simulink model "BLIMP_DYNAMICS_MODEL_HOLD"  (R2024b)
settings: Solver=VariableStepAuto  StartTime=0.0  StopTime=240  RelTol=1e-3
values from neighbouring files (symbols this model uses):
  A_alt_aug = [A_alt, zeros(size(A_alt,1),1); -C_alt, 0]    [ALTITUDE_DYNAMICS.m]
  A_fwd_aug = [A_fwd, zeros(size(A_fwd,1),1); -C_fwd, 0]    [FORWARD_DYNAMICS.m]
  A_rot_aug = [A_rot, zeros(size(A_rot,1),1); -C_rot, 0]    [ROTATIONAL_DYNAMICS.m]
  B_alt_aug = [B_alt; 0]    [ALTITUDE_DYNAMICS.m]
  B_fwd_aug = [B_fwd; 0]    [FORWARD_DYNAMICS.m]
  B_rot_aug = [B_rot; 0]    [ROTATIONAL_DYNAMICS.m]
  C_alt_aug = [C_alt 0]    [ALTITUDE_DYNAMICS.m]
  C_fwd_aug = [C_fwd 0]    [FORWARD_DYNAMICS.m]
  C_rot_aug = [C_rot 0]    [ROTATIONAL_DYNAMICS.m]
  D_alt_aug = D_alt    [ALTITUDE_DYNAMICS.m]
  D_fwd_aug = D_fwd    [FORWARD_DYNAMICS.m]
  D_rot_aug = D_rot    [ROTATIONAL_DYNAMICS.m]
  INIT_COND_alt = [0, 0, 0, 0]    [ALTITUDE_DYNAMICS.m]
  INIT_COND_fwd = [0, 0, 100, 0, 0]    [FORWARD_DYNAMICS.m]
  INIT_COND_rot = [0, 0, 0, 0]    [ROTATIONAL_DYNAMICS.m]
  q1_alt = 10    [ALTITUDE_DYNAMICS.m]
  q1_fwd = 0.1    [FORWARD_DYNAMICS.m]
  q1_rot = 10    [ROTATIONAL_DYNAMICS.m]
  q2_alt = 1    [ALTITUDE_DYNAMICS.m]
  q2_fwd = 1    [FORWARD_DYNAMICS.m]
  q2_rot = 100    [ROTATIONAL_DYNAMICS.m]
  q3_alt = 5    [ALTITUDE_DYNAMICS.m]
  q3_fwd = 5    [FORWARD_DYNAMICS.m]
  q3_rot = 1    [ROTATIONAL_DYNAMICS.m]
  q4_alt = 15    [ALTITUDE_DYNAMICS.m]
  q4_fwd = 5    [FORWARD_DYNAMICS.m]
  q4_rot = 100    [ROTATIONAL_DYNAMICS.m]
  q5_fwd = 10    [FORWARD_DYNAMICS.m]
  R_alt = 1    [ALTITUDE_DYNAMICS.m]
  R_fwd = 0.1    [FORWARD_DYNAMICS.m]
  R_rot = 0.01    [ROTATIONAL_DYNAMICS.m]
settings Model: Creator=hazza  LastModifiedBy=hazza

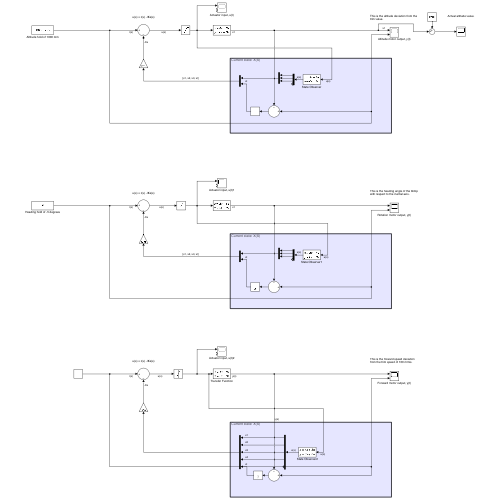
[thumbnail: Simulink's stored preview of the top-level diagram]
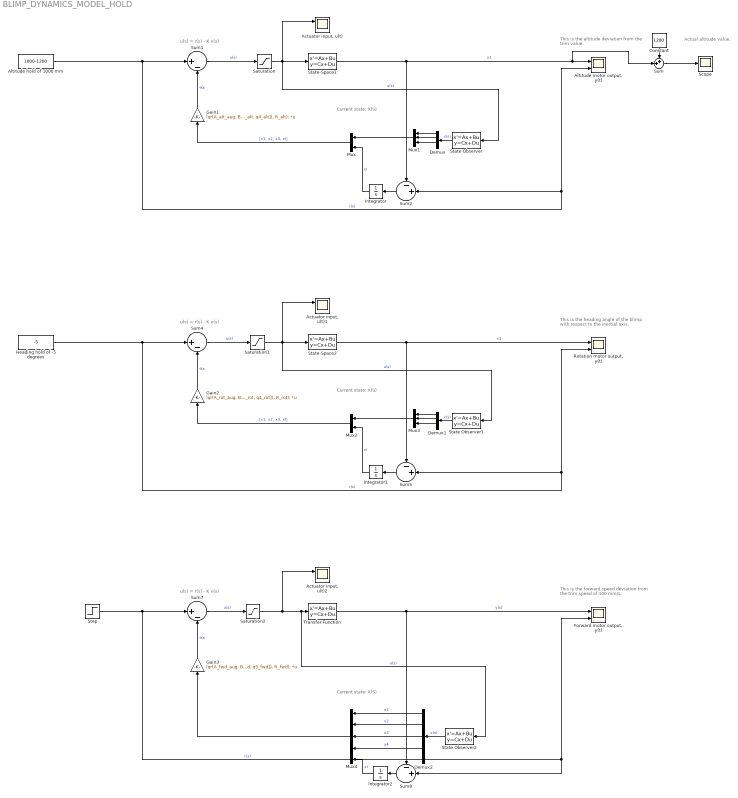
== system BLIMP_DYNAMICS_MODEL_HOLD ==
  note: u(s) = r(s) - K x(s)
  note: Current state: X(S)
  note: Current state: X(S)
  note: Current state: X(S)
  note: u(s) = r(s) - K x(s)
  note: u(s) = r(s) - K x(s)
  note: This is the forward speed deviation from the trim speed of 100 mm/s.
  note: This is the heading angle of the blimp with respect to the inertial axis.
  note: This is the altitude deviation from the trim value.
  note: Actual altitude value.
  "Actuator input, u(t)" : Scope  NumInputPorts=2
  "Actuator input, u(t)1" : Scope  NumInputPorts=2
  "Actuator input, u(t)2" : Scope  NumInputPorts=2
  Altitude hold of 1000 mm : Constant  Value=1000-1200
  "Altitude motor output, y(t)" : Scope  NumInputPorts=2
  Constant : Constant  Value=1200
  Demux : Demux
  Demux1 : Demux
  Demux2 : Demux  Outputs=5
  "Forward motor output, y(t)" : Scope  NumInputPorts=2
  Gain1 : Gain  Gain=lqr(A_alt_aug, B_alt_aug, diag([q1_alt, q2_alt, q3_alt, q4_alt]), R_alt);  Multiplication=Matrix(K*u)
  Gain2 : Gain  Gain=lqr(A_rot_aug, B_rot_aug, diag([q1_rot, q2_rot, q3_rot, q4_rot]), R_rot);  Multiplication=Matrix(K*u)
  Gain3 : Gain  Gain=lqr(A_fwd_aug, B_fwd_aug, diag([q1_fwd, q2_fwd, q3_fwd, q4_fwd, q5_fwd]), R_fwd);  Multiplication=Matrix(K*u)
  Heading hold of -5 degrees : Constant  Value=-5
  Integrator : Integrator
  Integrator1 : Integrator
  Integrator2 : Integrator
  Mux : Mux  Inputs=2
  Mux1 : Mux  Inputs=3
  Mux2 : Mux  Inputs=2
  Mux3 : Mux  Inputs=3
  Mux4 : Mux  Inputs=5
  "Rotation motor output, y(t)" : Scope  NumInputPorts=2
  Saturation : Saturate  UpperLimit=95  LowerLimit=-55  ZeroCross=off
  Saturation1 : Saturate  UpperLimit=150  LowerLimit=-150  ZeroCross=off
  Saturation2 : Saturate  UpperLimit=127  LowerLimit=-23  ZeroCross=off
  Scope : Scope
  State Observer : StateSpace  A=A_alt_aug  B=B_alt_aug  C=eye(4)  D=zeros(4,1)  InitialCondition=INIT_COND_alt
  State Observer1 : StateSpace  A=A_rot_aug  B=B_rot_aug  C=eye(4)  D=zeros(4,1)  InitialCondition=INIT_COND_rot
  State Observer2 : StateSpace  A=A_fwd_aug  B=B_fwd_aug  C=eye(5)  D=zeros(5,1)  InitialCondition=INIT_COND_fwd
  State-Space1 : StateSpace  A=A_alt_aug  B=B_alt_aug  C=C_alt_aug  D=D_alt_aug  InitialCondition=INIT_COND_alt
  State-Space2 : StateSpace  A=A_rot_aug  B=B_rot_aug  C=C_rot_aug  D=D_rot_aug  InitialCondition=INIT_COND_rot
  Step : Step  After=100  SampleTime=5
  Sum : Sum  Inputs=++|
  Sum1 : Sum  Inputs=|+-
  Sum2 : Sum  Inputs=-+|
  Sum4 : Sum  Inputs=|+-
  Sum5 : Sum  Inputs=-+|
  Sum7 : Sum  Inputs=|+-
  Sum8 : Sum  Inputs=-+|
  Transfer Function : StateSpace  A=A_fwd_aug  B=B_fwd_aug  C=C_fwd_aug  D=D_fwd_aug  InitialCondition=INIT_COND_fwd
  wires:
  Gain2/1 -> Sum4/2  "-Kx"
  Mux/1 -> Gain1/1  "[x1, x2, x3, xI]"
  Sum2/1 -> Integrator/1
  Demux1/1 -> Mux3/1
  Sum1/1 -> Saturation/1  "u(s)"
  Mux3/1 -> Mux2/1
  Altitude hold of 1000 mm/1 -> Sum1/1, "Altitude motor output, y(t)"/2, Sum2/2  "r(s)"
  Gain1/1 -> Sum1/2  "-Kx"
  Demux/1 -> Mux1/1
  Integrator1/1 -> Mux2/2  "xI"
  Demux/2 -> Mux1/2
  Sum5/1 -> Integrator1/1
  Saturation/1 -> State Observer/1, "Actuator input, u(t)"/1, State-Space1/1  "u(s)"
  Sum4/1 -> Saturation1/1  "u(s)"
  Mux4/1 -> Gain3/1
  State Observer1/1 -> Demux1/1  "x(s)"
  Demux1/3 -> Mux3/3
  Integrator2/1 -> Mux4/5  "xI"
  Demux2/1 -> Mux4/1  "x1"
  Demux2/4 -> Mux4/4  "x4"
  Sum8/1 -> Integrator2/1
  Step/1 -> Sum7/1, "Forward motor output, y(t)"/2, Sum8/2  "r(s)"
  Saturation2/1 -> State Observer2/1, Transfer Function/1, "Actuator input, u(t)2"/1  "u(s)"
  Demux2/2 -> Mux4/2  "x2"
  State-Space2/1 -> Sum5/1, "Rotation motor output, y(t)"/1  "x1"
  State Observer2/1 -> Demux2/1  "x(s)"
  Demux2/3 -> Mux4/3  "x3"
  Mux1/1 -> Mux/1
  State Observer/1 -> Demux/1  "x(s)"
  Mux2/1 -> Gain2/1  "[x1, x2, x3, xI]"
  Saturation1/1 -> "Actuator input, u(t)1"/1, State Observer1/1, State-Space2/1  "u(s)"
  Demux1/2 -> Mux3/2
  Transfer Function/1 -> "Forward motor output, y(t)"/1, Sum8/1  "y(s)"
  Demux/3 -> Mux1/3
  Gain3/1 -> Sum7/2  "-Kx"
  Heading hold of -5 degrees/1 -> Sum4/1, "Rotation motor output, y(t)"/2, Sum5/2  "r(s)"
  Integrator/1 -> Mux/2  "xI"
  State-Space1/1 -> Sum2/1, Sum/2, "Altitude motor output, y(t)"/1  "x1"
  Sum7/1 -> Saturation2/1  "u(s)"
  Constant/1 -> Sum/1
  Sum/1 -> Scope/1
